simulink model "modelos_lti_simp_y_aum_para_informe"  (R2019a)
settings: Solver=VariableStepAuto  StartTime=0.0  StopTime=10.0  RelTol=1e-3
undefined symbols (not defined in the file): b_eq, J_eq, L_d, L_q, lambda_m, P_p, r, R_s_prom
settings Model: Creator=pedro  LastModifiedBy=pedro

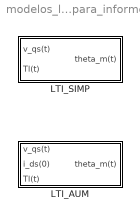
== system modelos_lti_simp_y_aum_para_informe ==
  LTI_AUM : Subsystem
  LTI_SIMP : Subsystem

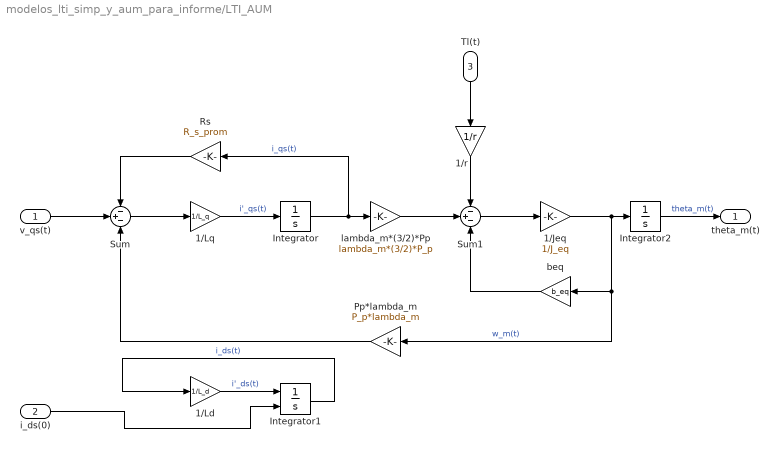
== system modelos_lti_simp_y_aum_para_informe/LTI_AUM ==
  v_qs(t) : Inport
  i_ds(0) : Inport  Port=2
  Tl(t) : Inport  Port=3
  1/Jeq : Gain  Gain=1/J_eq
  1/Ld : Gain  Gain=1/L_d
  1/Lq : Gain  Gain=1/L_q
  1/r : Gain  Gain=1/r
  Integrator : Integrator
  Integrator1 : Integrator  InitialConditionSource=external
  Integrator2 : Integrator
  Pp*lambda_m : Gain  Gain=P_p*lambda_m
  Rs : Gain  Gain=R_s_prom
  Sum : Sum  Inputs=-+-
  Sum1 : Sum  Inputs=-+-
  beq : Gain  Gain=b_eq
  lambda_m*(3/2)*Pp : Gain  Gain=lambda_m*(3/2)*P_p
  theta_m(t) : Outport
  wires:
  1/Jeq/1 -> Integrator2/1, beq/1, Pp*lambda_m/1  "w_m(t)"
  Integrator/1 -> Rs/1, lambda_m*(3/2)*Pp/1  "i_qs(t)"
  Tl(t)/1 -> 1/r/1
  v_qs(t)/1 -> Sum/2
  1/r/1 -> Sum1/1
  beq/1 -> Sum1/3
  Rs/1 -> Sum/1
  1/Lq/1 -> Integrator/1  "i'_qs(t)"
  Sum1/1 -> 1/Jeq/1
  lambda_m*(3/2)*Pp/1 -> Sum1/2
  Sum/1 -> 1/Lq/1
  Pp*lambda_m/1 -> Sum/3
  1/Ld/1 -> Integrator1/1  "i'_ds(t)"
  Integrator1/1 -> 1/Ld/1  "i_ds(t)"
  i_ds(0)/1 -> Integrator1/2
  Integrator2/1 -> theta_m(t)/1  "theta_m(t)"

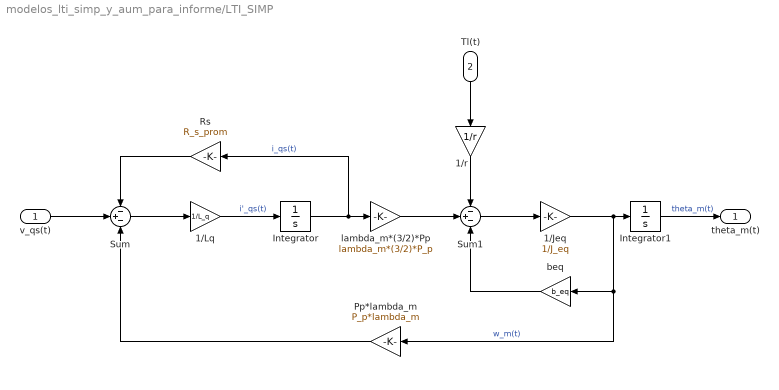
== system modelos_lti_simp_y_aum_para_informe/LTI_SIMP ==
  v_qs(t) : Inport
  Tl(t) : Inport  Port=2
  1/Jeq : Gain  Gain=1/J_eq
  1/Lq : Gain  Gain=1/L_q
  1/r : Gain  Gain=1/r
  Integrator : Integrator
  Integrator1 : Integrator
  Pp*lambda_m : Gain  Gain=P_p*lambda_m
  Rs : Gain  Gain=R_s_prom
  Sum : Sum  Inputs=-+-
  Sum1 : Sum  Inputs=-+-
  beq : Gain  Gain=b_eq
  lambda_m*(3/2)*Pp : Gain  Gain=lambda_m*(3/2)*P_p
  theta_m(t) : Outport
  wires:
  1/Jeq/1 -> Integrator1/1, beq/1, Pp*lambda_m/1  "w_m(t)"
  Integrator/1 -> Rs/1, lambda_m*(3/2)*Pp/1  "i_qs(t)"
  Tl(t)/1 -> 1/r/1
  v_qs(t)/1 -> Sum/2
  1/r/1 -> Sum1/1
  beq/1 -> Sum1/3
  Rs/1 -> Sum/1
  1/Lq/1 -> Integrator/1  "i'_qs(t)"
  Sum1/1 -> 1/Jeq/1
  lambda_m*(3/2)*Pp/1 -> Sum1/2
  Sum/1 -> 1/Lq/1
  Pp*lambda_m/1 -> Sum/3
  Integrator1/1 -> theta_m(t)/1  "theta_m(t)"
